simulink model "Exercise_2"  (R2022a)
settings: Solver=VariableStepAuto  StartTime=0.0  StopTime=10.0  RelTol=1e-3
settings Model: Creator=Shocky  LastModifiedBy=Shocky

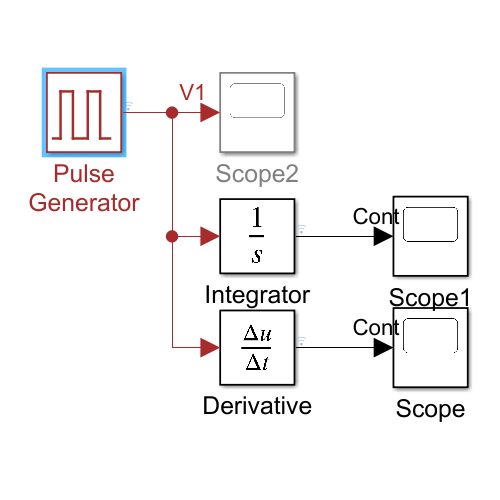
[thumbnail: Simulink's stored preview of the top-level diagram]
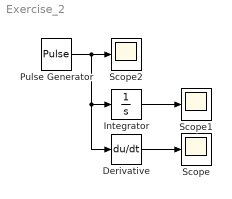
== system Exercise_2 ==
  Derivative : Derivative
  Integrator : Integrator
  Pulse Generator : DiscretePulseGenerator  PulseType=Time based  Amplitude=10  Period=10  PulseWidth=5
  Scope : Scope
  Scope1 : Scope
  Scope2 : Scope
  wires:
  Integrator/1 -> Scope1/1
  Derivative/1 -> Scope/1
  Pulse Generator/1 -> Integrator/1, Derivative/1, Scope2/1
